simulink model "ass7measurements"  (R2018a)
settings: Solver=VariableStepAuto  StartTime=0.0  StopTime=10.0  RelTol=1e-3
settings Model: Creator=arjun  LastModifiedBy=arjun

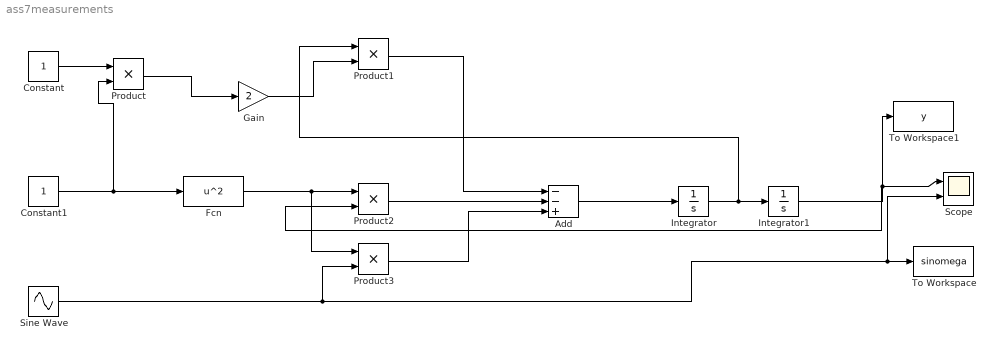
== system ass7measurements ==
  Add : Sum  Inputs=--+
  Constant : Constant
  Constant1 : Constant
  Fcn : Fcn  Expr=u^2
  Gain : Gain  Gain=2
  Integrator : Integrator
  Integrator1 : Integrator
  Product{,1..3} (4 alike) : Product
  Scope : Scope  NumInputPorts=2
  Sine Wave : Sin  SampleTime=0
  To Workspace : ToWorkspace  VariableName=sinomega  SaveFormat=Timeseries  SampleTime=-1
  To Workspace1 : ToWorkspace  VariableName=y  SaveFormat=Timeseries  SampleTime=-1
  wires:
  Constant/1 -> Product/1
  Constant1/1 -> Product/2, Fcn/1
  Product/1 -> Gain/1
  Gain/1 -> Product1/2
  Product1/1 -> Add/1
  Product2/1 -> Add/2
  Product3/1 -> Add/3
  Fcn/1 -> Product3/1, Product2/1
  Add/1 -> Integrator/1
  Integrator/1 -> Product1/1, Integrator1/1
  Integrator1/1 -> Product2/2, Scope/1, To Workspace1/1
  Sine Wave/1 -> Product3/2, Scope/2, To Workspace/1
